simulink model "total_senario"  (R2019a)
settings: Solver=ode4  StartTime=0.0  StopTime=40  FixedStep=0.001  RelTol=1e-3
libraries: nesl_utility x16, sm_lib x13, simulink x1
(part 1 of 3)
settings Model: Creator=spring  LastModifiedBy=spring-dorosee

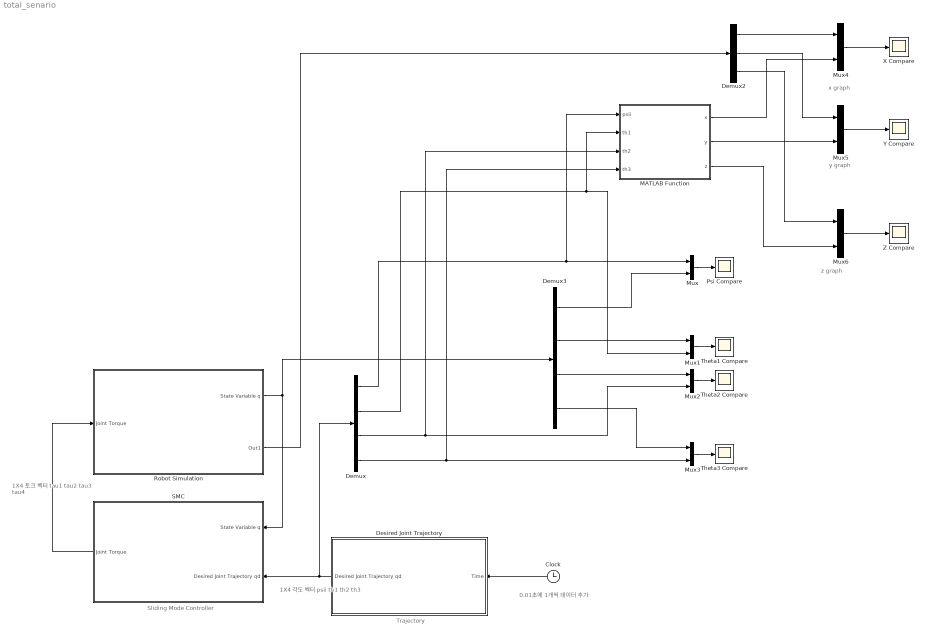
== system total_senario ==
  note: z graph
  note: y graph
  note: x graph
  note: 1X4 각도 벡터
      | psii
      | th1
      | th2
      | th3
  note: 0.01초에 1개씩 데이터 추가
  note: Trajectory
  note: Sliding Mode Controller
  note: 1X4 토크 벡터
      | tau1
      | tau2
      | tau3
      | tau4
  Clock : Clock
  Demux : Demux
  Demux2 : Demux  Outputs=3
  Demux3 : Demux
  Desired Joint Trajectory : Subsystem
  MATLAB Function : MATLAB Function  TreatAsAtomicUnit=on
  Mux{,1..6} (7 alike) : Mux  Inputs=2
  Psi Compare : Scope
  Robot Simulation : Subsystem
  SMC : Subsystem
  Theta1 Compare : Scope
  Theta2 Compare : Scope
  Theta3 Compare : Scope
  X Compare : Scope
  Y Compare : Scope
  Z Compare : Scope
  wires:
  SMC/1(Joint Torque) -> Robot Simulation/1(Joint Torque)
  Robot Simulation/1(State Variable q) -> SMC/1(State Variable q), Demux3/1
  Demux/1 -> MATLAB Function/1(psii), Mux/1
  Demux/2 -> Mux1/2, MATLAB Function/2(th1)
  Demux/3 -> Mux2/2, MATLAB Function/3(th2)
  Demux/4 -> Mux3/2, MATLAB Function/4(th3)
  Clock/1 -> Desired Joint Trajectory/1(Time)
  Desired Joint Trajectory/1(Desired Joint Trajectory qd) -> SMC/2(Desired Joint Trajectory qd), Demux/1
  Demux3/1 -> Mux/2
  Demux3/2 -> Mux1/1
  Demux3/3 -> Mux2/1
  Demux3/4 -> Mux3/1
  Mux/1 -> Psi Compare/1
  Mux1/1 -> Theta1 Compare/1
  Mux3/1 -> Theta3 Compare/1
  Mux2/1 -> Theta2 Compare/1
  Robot Simulation/2(Out1) -> Demux2/1
  Demux2/1 -> Mux4/1
  Demux2/2 -> Mux5/1
  MATLAB Function/1(x) -> Mux4/2
  MATLAB Function/2(y) -> Mux5/2
  Mux5/1 -> Y Compare/1
  Mux4/1 -> X Compare/1
  Demux2/3 -> Mux6/1
  MATLAB Function/3(z) -> Mux6/2
  Mux6/1 -> Z Compare/1

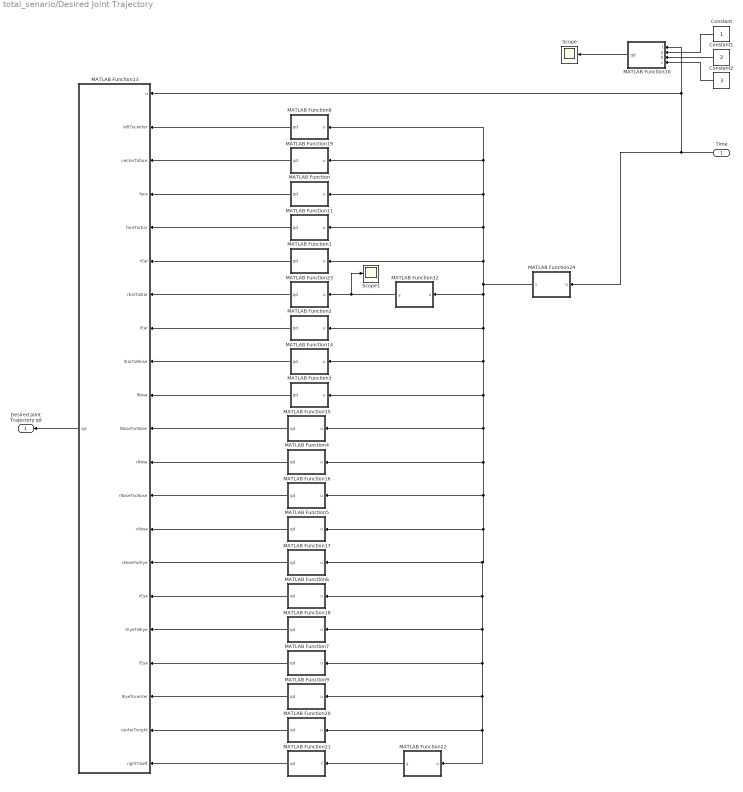
== system total_senario/Desired Joint Trajectory ==
  Time : Inport
  Constant : Constant
  Constant1 : Constant  Value=2
  Constant2 : Constant  Value=3
  MATLAB Function : MATLAB Function  TreatAsAtomicUnit=on
  MATLAB Function1 : MATLAB Function  TreatAsAtomicUnit=on
  MATLAB Function10 : MATLAB Function  TreatAsAtomicUnit=on
  MATLAB Function11 : MATLAB Function  TreatAsAtomicUnit=on
  MATLAB Function12 : MATLAB Function  TreatAsAtomicUnit=on
  MATLAB Function13 : MATLAB Function  TreatAsAtomicUnit=on
  MATLAB Function14 : MATLAB Function  TreatAsAtomicUnit=on
  MATLAB Function15 : MATLAB Function  TreatAsAtomicUnit=on
  MATLAB Function16 : MATLAB Function  TreatAsAtomicUnit=on
  MATLAB Function17 : MATLAB Function  TreatAsAtomicUnit=on
  MATLAB Function18 : MATLAB Function  TreatAsAtomicUnit=on
  MATLAB Function19 : MATLAB Function  TreatAsAtomicUnit=on
  MATLAB Function2 : MATLAB Function  TreatAsAtomicUnit=on
  MATLAB Function20 : MATLAB Function  TreatAsAtomicUnit=on
  MATLAB Function21 : MATLAB Function  TreatAsAtomicUnit=on
  MATLAB Function22 : MATLAB Function  TreatAsAtomicUnit=on
  MATLAB Function23 : MATLAB Function  TreatAsAtomicUnit=on
  MATLAB Function24 : MATLAB Function  TreatAsAtomicUnit=on
  MATLAB Function3 : MATLAB Function  TreatAsAtomicUnit=on
  MATLAB Function4 : MATLAB Function  TreatAsAtomicUnit=on
  MATLAB Function5 : MATLAB Function  TreatAsAtomicUnit=on
  MATLAB Function6 : MATLAB Function  TreatAsAtomicUnit=on
  MATLAB Function7 : MATLAB Function  TreatAsAtomicUnit=on
  MATLAB Function8 : MATLAB Function  TreatAsAtomicUnit=on
  MATLAB Function9 : MATLAB Function  TreatAsAtomicUnit=on
  Scope : Scope
  Scope1 : Scope
  Desired Joint Trajectory qd : Outport
  wires:
  MATLAB Function13/1(qd) -> Desired Joint Trajectory qd/1
  MATLAB Function10/1(qd) -> Scope/1
  Constant/1 -> MATLAB Function10/2(a)
  Constant1/1 -> MATLAB Function10/3(b)
  Constant2/1 -> MATLAB Function10/4(c)
  MATLAB Function19/1(qd) -> MATLAB Function13/3(centerToface)
  MATLAB Function/1(qd) -> MATLAB Function13/4(face)
  MATLAB Function11/1(qd) -> MATLAB Function13/5(faceTorEar)
  MATLAB Function1/1(qd) -> MATLAB Function13/6(rEar)
  MATLAB Function2/1(qd) -> MATLAB Function13/8(lEar)
  MATLAB Function14/1(qd) -> MATLAB Function13/9(lEarTolNose)
  MATLAB Function3/1(qd) -> MATLAB Function13/10(lNose)
  MATLAB Function15/1(qd) -> MATLAB Function13/11(lNoseTorNose)
  MATLAB Function4/1(qd) -> MATLAB Function13/12(rNose)
  MATLAB Function16/1(qd) -> MATLAB Function13/13(rNoseTocNose)
  MATLAB Function5/1(qd) -> MATLAB Function13/14(cNose)
  MATLAB Function17/1(qd) -> MATLAB Function13/15(cNoseTorEye)
  MATLAB Function6/1(qd) -> MATLAB Function13/16(rEye)
  MATLAB Function18/1(qd) -> MATLAB Function13/17(rEyeTolEye)
  MATLAB Function7/1(qd) -> MATLAB Function13/18(lEye)
  MATLAB Function8/1(qd) -> MATLAB Function13/2(leftTocenter)
  MATLAB Function9/1(qd) -> MATLAB Function13/19(lEyeTocenter)
  MATLAB Function20/1(qd) -> MATLAB Function13/20(centerToright)
  MATLAB Function21/1(qd) -> MATLAB Function13/21(rightToleft)
  MATLAB Function23/1(qd) -> MATLAB Function13/7(rEarTolEar)
  MATLAB Function12/1(y) -> Scope1/1, MATLAB Function23/1(u)
  MATLAB Function22/1(y) -> MATLAB Function21/1(t)
  Time/1 -> MATLAB Function24/1(u), MATLAB Function13/1(u), MATLAB Function10/1(t)
  MATLAB Function24/1(s) -> MATLAB Function1/1(u), MATLAB Function11/1(u), MATLAB Function/1(u), MATLAB Function19/1(u), MATLAB Function8/1(u), MATLAB Function22/1(u), MATLAB Function20/1(u), MATLAB Function9/1(u), MATLAB Function7/1(u), MATLAB Function18/1(u), MATLAB Function6/1(u), MATLAB Function17/1(u), MATLAB Function5/1(u), MATLAB Function16/1(u), MATLAB Function4/1(u), MATLAB Function15/1(u), MATLAB Function3/1(u), MATLAB Function14/1(u), MATLAB Function2/1(u), MATLAB Function12/1(u)

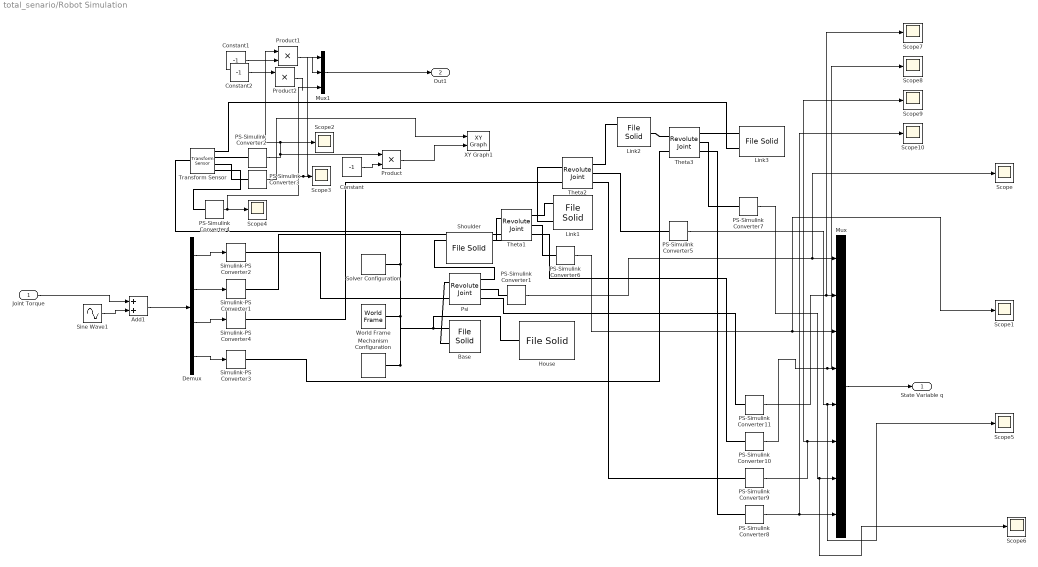
== system total_senario/Robot Simulation ==
  Joint Torque : Inport
  Add1 : Sum
  Base : sm_lib/Body Elements/File Solid  ExtGeomFileName=/Users/spring-dorosee/Desktop/project/inha/2학년 부분학기/로봇공학/로보트롤스/modeling/RotateBase.step  UnitType=FromFile  ExtGeomFileUnits=m  InertiaType=CalculateFromGeometry  Mass=2.945  MassUnits=kg  CenterOfMass=[0 0 0]  CenterOfMassUnits=m  MomentsOfInertia=[1 1 1]  MomentsOfInertiaUnits=kg*m^2  ProductsOfInertia=[0 0 0]  ProductsOfInertiaUnits=kg*m^2  BasedOnType=Density  Density=1000  DensityUnits=kg/m^3  DoExposeReferenceFrame=on  SerializedFrames=<Frames><Frame><Id>Frame1</Id><Value><Name>BaseFrame</Name><Origin><Source>GeometricFeature</Source><FeatureName>planar surface 2</FeatureName></Origin><PrimaryAxis><DefinedDirection>+Z</DefinedDirection><Source>ReferenceFrame</Source><SourceDirection>+Z</SourceDirection><FeatureName></FeatureName></PrimaryAxis><SecondaryAxis><DefinedDirection>+X</DefinedDirection><Source>ReferenceFrame</Source><SourceDirection>+X</SourceDirection><FeatureName></FeatureName></SecondaryAxis></Value></Frame><Frame><Id>Frame2</Id><Value><Name>Shoulder</Name><Origin><Source>GeometricFeature</Source><FeatureName>planar surface 1</FeatureName></Origin><PrimaryAxis><DefinedDirection>+Z</DefinedDirection><Source>ReferenceFrame</Source><SourceDirection>+Z</SourceDirection><FeatureName></FeatureName></PrimaryAxis><SecondaryAxis><DefinedDirection>+X</DefinedDirection><Source>ReferenceFrame</Source><SourceDirection>+X</SourceDirection><FeatureName></FeatureName></SecondaryAxis></Value></Frame></Frames>  GraphicType=FromGeometry  MarkerShape=Sphere  MarkerSize=10  GraphicVisPropType=SimpleVisualProperties  GraphicDiffuseColor=[0.0 0.8 0.8]  GraphicSpecularColor=[0.5 0.5 0.5 1.0]  GraphicAmbientColor=[0.15 0.15 0.15 1.0]  GraphicEmissiveColor=[0.0 0.0 0.0 1.0]  GraphicShininess=75  GraphicOpacity=1.0
  Constant : Constant  Value=-1
  Constant1 : Constant  Value=-1
  Constant2 : Constant  Value=-1
  Demux : Demux
  House : sm_lib/Body Elements/File Solid  ExtGeomFileName=C:\Users\Hyeong Deok Seo\Desktop\robot_matlab\deok\robot_team\simul\house.step  UnitType=FromFile  ExtGeomFileUnits=m  InertiaType=Custom  Mass=0.1  MassUnits=kg  CenterOfMass=[0 0 0.08]  CenterOfMassUnits=m  MomentsOfInertia=[1 1 1]  MomentsOfInertiaUnits=kg*m^2  ProductsOfInertia=[0 0 0]  ProductsOfInertiaUnits=kg*m^2  BasedOnType=Density  Density=1000  DensityUnits=kg/m^3  DoExposeReferenceFrame=off  SerializedFrames=<Frames><Frame><Id>Frame1</Id><Value><Name>BaseFrame</Name><Origin><Source>GeometricFeature</Source><FeatureName>planar surface 7</FeatureName></Origin><PrimaryAxis><DefinedDirection>+Z</DefinedDirection><Source>ReferenceFrame</Source><SourceDirection>+Z</SourceDirection><FeatureName></FeatureName></PrimaryAxis><SecondaryAxis><DefinedDirection>+X</DefinedDirection><Source>GeometricFeature</Source><SourceDirection>+X</SourceDirection><FeatureName>planar surface 4</FeatureName></SecondaryAxis></Value></Frame></Frames>  GraphicType=FromGeometry  MarkerShape=Sphere  MarkerSize=10  GraphicVisPropType=SimpleVisualProperties  GraphicDiffuseColor=[1.0 1.0 0.2]  GraphicSpecularColor=[0.5 0.5 0.5 1.0]  GraphicAmbientColor=[0.15 0.15 0.15 1.0]  GraphicEmissiveColor=[0.0 0.0 0.0 1.0]  GraphicShininess=75  GraphicOpacity=1.0
  Link1 : sm_lib/Body Elements/File Solid  ExtGeomFileName=/Users/spring-dorosee/Desktop/project/inha/2학년 부분학기/로봇공학/로보트롤스/modeling/link1_30cm.step  UnitType=FromFile  ExtGeomFileUnits=m  InertiaType=Custom  Mass=4  MassUnits=kg  CenterOfMass=[0 0 0.38]  CenterOfMassUnits=m  MomentsOfInertia=[0 0 0]  MomentsOfInertiaUnits=kg*m^2  ProductsOfInertia=[0 0 0]  ProductsOfInertiaUnits=kg*m^2  BasedOnType=Density  Density=1000  DensityUnits=kg/m^3  DoExposeReferenceFrame=on  SerializedFrames=<Frames><Frame><Id>Frame1</Id><Value><Name>Theta1</Name><Origin><Source>GeometricFeature</Source><FeatureName>planar surface 2</FeatureName></Origin><PrimaryAxis><DefinedDirection>+X</DefinedDirection><Source>ReferenceFrame</Source><SourceDirection>+Z</SourceDirection><FeatureName></FeatureName></PrimaryAxis><SecondaryAxis><DefinedDirection>+Z</DefinedDirection><Source>ReferenceFrame</Source><SourceDirection>+X</SourceDirection><FeatureName></FeatureName></SecondaryAxis></Value></Frame><Frame><Id>Frame2</Id><Value><Name>Theta2</Name><Origin><Source>CenterOfMassFrame</Source><FeatureName></FeatureName></Origin><PrimaryAxis><DefinedDirection>+X</DefinedDirection><Source>ReferenceFrame</Source><SourceDirection>+Z</SourceDirection><FeatureName></FeatureName></PrimaryAxis><SecondaryAxis><DefinedDirection>+Z</DefinedDirection><Source>ReferenceFrame</Source><SourceDirection>+X</SourceDirection><FeatureName></FeatureName></SecondaryAxis></Value></Frame></Frames>  GraphicType=FromGeometry  MarkerShape=Sphere  MarkerSize=10  GraphicVisPropType=SimpleVisualProperties  GraphicDiffuseColor=[0.6 0.6 1.0]  GraphicSpecularColor=[0.5 0.5 0.5 1.0]  GraphicAmbientColor=[0.15 0.15 0.15 1.0]  GraphicEmissiveColor=[0.0 0.0 0.0 1.0]  GraphicShininess=75  GraphicOpacity=1.0
  Link2 : sm_lib/Body Elements/File Solid  ExtGeomFileName=/Users/spring-dorosee/Desktop/project/inha/2학년 부분학기/로봇공학/로보트롤스/modeling/link1_30cm.step  UnitType=FromFile  ExtGeomFileUnits=m  InertiaType=Custom  Mass=3  MassUnits=kg  CenterOfMass=[0 0 0.38]  CenterOfMassUnits=m  MomentsOfInertia=[0 0 0]  MomentsOfInertiaUnits=kg*m^2  ProductsOfInertia=[0 0 0]  ProductsOfInertiaUnits=kg*m^2  BasedOnType=Density  Density=1000  DensityUnits=kg/m^3  DoExposeReferenceFrame=off  SerializedFrames=<Frames><Frame><Id>Frame1</Id><Value><Name>Theta2</Name><Origin><Source>GeometricFeature</Source><FeatureName>planar surface 2</FeatureName></Origin><PrimaryAxis><DefinedDirection>+X</DefinedDirection><Source>ReferenceFrame</Source><SourceDirection>+Z</SourceDirection><FeatureName></FeatureName></PrimaryAxis><SecondaryAxis><DefinedDirection>+Z</DefinedDirection><Source>ReferenceFrame</Source><SourceDirection>+X</SourceDirection><FeatureName></FeatureName></SecondaryAxis></Value></Frame><Frame><Id>Frame2</Id><Value><Name>Theta3</Name><Origin><Source>CenterOfMassFrame</Source><FeatureName></FeatureName></Origin><PrimaryAxis><DefinedDirection>+X</DefinedDirection><Source>ReferenceFrame</Source><SourceDirection>+Z</SourceDirection><FeatureName></FeatureName></PrimaryAxis><SecondaryAxis><DefinedDirection>+Z</DefinedDirection><Source>ReferenceFrame</Source><SourceDirection>+X</SourceDirection><FeatureName></FeatureName></SecondaryAxis></Value></Frame><Frame><Id>Frame3</Id><Value><Name>XYZ</Name><Origin><Source>GeometricFeature</Source><FeatureName>cylindrical surface 7</FeatureName></Origin><PrimaryAxis><DefinedDirection>+X</DefinedDirection><Source>ReferenceFrame</Source><SourceDirection>+Z</SourceDirection><FeatureName></FeatureName></PrimaryAxis><SecondaryAxis><DefinedDirection>+Z</DefinedDirection><Source>ReferenceFrame</Source><SourceDirection>+X</SourceDirection><FeatureName></FeatureName></SecondaryAxis></Value></Frame></Frames>  GraphicType=FromGeometry  MarkerShape=Sphere  MarkerSize=10  GraphicVisPropType=SimpleVisualProperties  GraphicDiffuseColor=[1.0 0.6 0.6]  GraphicSpecularColor=[0.5 0.5 0.5 1.0]  GraphicAmbientColor=[0.15 0.15 0.15 1.0]  GraphicEmissiveColor=[0.0 0.0 0.0 1.0]  GraphicShininess=75  GraphicOpacity=1.0
  Link3 : sm_lib/Body Elements/File Solid  ExtGeomFileName=/Users/spring-dorosee/Desktop/project/inha/2학년 부분학기/로봇공학/로보트롤스/modeling/WafflePlate.step  UnitType=FromFile  ExtGeomFileUnits=m  InertiaType=Custom  Mass=1  MassUnits=kg  CenterOfMass=[0 0 0.856]  CenterOfMassUnits=m  MomentsOfInertia=[0 0 0]  MomentsOfInertiaUnits=kg*m^2  ProductsOfInertia=[0 0 0]  ProductsOfInertiaUnits=kg*m^2  BasedOnType=Density  Density=1000  DensityUnits=kg/m^3  DoExposeReferenceFrame=on  SerializedFrames=<Frames><Frame><Id>Frame1</Id><Value><Name>Theta3</Name><Origin><Source>GeometricFeature</Source><FeatureName>planar surface 1</FeatureName></Origin><PrimaryAxis><DefinedDirection>+X</DefinedDirection><Source>ReferenceFrame</Source><SourceDirection>+Z</SourceDirection><FeatureName></FeatureName></PrimaryAxis><SecondaryAxis><DefinedDirection>+Z</DefinedDirection><Source>ReferenceFrame</Source><SourceDirection>+X</SourceDirection><FeatureName></FeatureName></SecondaryAxis></Value></Frame><Frame><Id>Frame2</Id><Value><Name>CenterMass</Name><Origin><Source>CenterOfMassFrame</Source><FeatureName></FeatureName></Origin><PrimaryAxis><DefinedDirection>+Z</DefinedDirection><Source>ReferenceFrame</Source><SourceDirection>+Z</SourceDirection><FeatureName></FeatureName></PrimaryAxis><SecondaryAxis><DefinedDirection>+X</DefinedDirection><Source>ReferenceFrame</Source><SourceDirection>+X</SourceDirection><FeatureName></FeatureName></SecondaryAxis></Value></Frame></Frames>  GraphicType=FromGeometry  MarkerShape=Sphere  MarkerSize=10  GraphicVisPropType=SimpleVisualProperties  GraphicDiffuseColor=[0.4 1.0 0.4]  GraphicSpecularColor=[0.5 0.5 0.5 1.0]  GraphicAmbientColor=[0.15 0.15 0.15 1.0]  GraphicEmissiveColor=[0.0 0.0 0.0 1.0]  GraphicShininess=75  GraphicOpacity=1.0
  Mechanism Configuration : sm_lib/Utilities/Mechanism Configuration  UniformGravity=Constant  GravityVector=[0 0 -9.81]  GravityUnits=m/s^2  LinearizationDelta=0.001
  Mux : Mux  Inputs=8
  Mux1 : Mux  Inputs=3
  PS-Simulink Converter{1..11} (11 alike) : nesl_utility/PS-Simulink Converter  PhysicalDomain=network_engine_domain  SubClassName=ps_output  LeftPortType=input  RightPortType=output  PseudoPeriodic=off  Frequencies=[]  Unit=1  AffineConversion=off
      settings: SourceProductBaseCode=PW,SS
  Product : Product
  Product1 : Product
  Product2 : Product
  Psi : sm_lib/Joints/Revolute Joint  SenseConstraintForce=off  SenseConstraintForceX=off  SenseConstraintForceY=off  SenseConstraintForceZ=off  SenseConstraintTorque=off  SenseConstraintTorqueX=off  SenseConstraintTorqueY=off  SenseConstraintTorqueZ=off  SenseTotalForce=off  SenseTotalForceX=off  SenseTotalForceY=off  SenseTotalForceZ=off  SenseTotalTorque=off  SenseTotalTorqueX=off  SenseTotalTorqueY=off  SenseTotalTorqueZ=off  CompositeWrenchDir=FollowerOnBase  CompositeWrenchFrame=BaseFrame  EquilibriumPosition=0  EquilibriumPositionUnits=deg  SpringStiffness=0  SpringStiffnessUnits=N*m/deg  DampingCoefficient=0  DampingCoefficientUnits=N*m/(deg/s)  TorqueActuationMode=InputTorque  MotionActuationMode=ComputedMotion  SensePosition=on  SenseVelocity=on  SenseAcceleration=off  SenseTorqueForce=off  SenseLowerLimitTorqueForce=off  SenseUpperLimitTorqueForce=off  LowerLimitSpecify=off  LowerLimitBound=-90  LowerLimitBoundUnits=deg  LowerLimitStiffness=1e4  LowerLimitStiffnessUnits=N*m/deg  LowerLimitDamping=10  LowerLimitDampingUnits=N*m/(deg/s)  LowerLimitTransitionRegionWidth=0.1  LowerLimitTransitionRegionWidthUnits=deg  UpperLimitSpecify=off  UpperLimitBound=90  UpperLimitBoundUnits=deg  UpperLimitStiffness=1e4  UpperLimitStiffnessUnits=N*m/deg  UpperLimitDamping=10  UpperLimitDampingUnits=N*m/(deg/s)  UpperLimitTransitionRegionWidth=0.1  UpperLimitTransitionRegionWidthUnits=deg  PositionTargetSpecify=on  PositionTargetPriority=High  PositionTargetValue=2.3562  PositionTargetValueUnits=rad  VelocityTargetSpecify=on  VelocityTargetPriority=High  VelocityTargetValue=0  VelocityTargetValueUnits=deg/s
  Scope{,1..10} (11 alike) : Scope
  Shoulder : sm_lib/Body Elements/File Solid  ExtGeomFileName=/Users/spring-dorosee/Desktop/project/inha/2학년 부분학기/로봇공학/로보트롤스/modeling/Shoulder.step  UnitType=FromFile  ExtGeomFileUnits=m  InertiaType=Custom  Mass=500  MassUnits=kg  CenterOfMass=[0 0 0.08]  CenterOfMassUnits=m  MomentsOfInertia=[0 0 0]  MomentsOfInertiaUnits=kg*m^2  ProductsOfInertia=[0 0 0]  ProductsOfInertiaUnits=kg*m^2  BasedOnType=Density  Density=1000  DensityUnits=kg/m^3  DoExposeReferenceFrame=on  SerializedFrames=<Frames><Frame><Id>Frame1</Id><Value><Name>Theta1</Name><Origin><Source>CenterOfMassFrame</Source><FeatureName></FeatureName></Origin><PrimaryAxis><DefinedDirection>+Y</DefinedDirection><Source>ReferenceFrame</Source><SourceDirection>+Z</SourceDirection><FeatureName></FeatureName></PrimaryAxis><SecondaryAxis><DefinedDirection>+Z</DefinedDirection><Source>ReferenceFrame</Source><SourceDirection>+X</SourceDirection><FeatureName></FeatureName></SecondaryAxis></Value></Frame><Frame><Id>Frame2</Id><Value><Name>ShoulderFrame</Name><Origin><Source>CenterOfMassFrame</Source><FeatureName></FeatureName></Origin><PrimaryAxis><DefinedDirection>+Z</DefinedDirection><Source>ReferenceFrame</Source><SourceDirection>+Z</SourceDirection><FeatureName></FeatureName></PrimaryAxis><SecondaryAxis><DefinedDirection>+X</DefinedDirection><Source>ReferenceFrame</Source><SourceDirection>+X</SourceDirection><FeatureName></FeatureName></SecondaryAxis></Value></Frame><Frame><Id>Frame3</Id><Value><Name>F3</Name><Origin><Source>CenterOfMassFrame</Source><FeatureName></FeatureName></Origin><PrimaryAxis><DefinedDirection>+Z</DefinedDirection><Source>ReferenceFrame</Source><SourceDirection>+Z</SourceDirection><FeatureName></FeatureName></PrimaryAxis><SecondaryAxis><DefinedDirection>+X</DefinedDirection><Source>ReferenceFrame</Source><SourceDirection>+X</SourceDirection><FeatureName></FeatureName></SecondaryAxis></Value></Frame></Frames>  GraphicType=FromGeometry  MarkerShape=Sphere  MarkerSize=10  GraphicVisPropType=SimpleVisualProperties  GraphicDiffuseColor=[1.0 1.0 0.2]  GraphicSpecularColor=[0.5 0.5 0.5 1.0]  GraphicAmbientColor=[0.15 0.15 0.15 1.0]  GraphicEmissiveColor=[0.0 0.0 0.0 1.0]  GraphicShininess=75  GraphicOpacity=1.0
  Simulink-PS Converter{1..4} (4 alike) : nesl_utility/Simulink-PS Converter  PhysicalDomain=network_engine_domain  SubClassName=ps_input  LeftPortType=input  RightPortType=output  PseudoPeriodic=off  Frequencies=[]  NoiseDistribution=none  NoiseParameters=[]  Unit=1  AffineConversion=off  FilteringAndDerivatives=filter  SimscapeFilterOrder=2  InputFilterTimeConstant=0.001  UdotUserProvided=1
      settings: SourceProductBaseCode=PW,SS
  Sine Wave1 : Sin  Amplitude=0.1  SampleTime=0
  Solver Configuration : nesl_utility/Solver Configuration  PhysicalDomain=network_engine_domain  SubClassName=solver  LeftPortType=input  RightPortType=generic  Tones=[]  Harmonics=[]  SimulateNoise=off  Profile=off  UseLocalSampling=off  EnableSwitchedLinearOptims=on  FrequencyDomain=off  UseCCode=off  RelTol=0.001  AbsTol=1e-06  MinStep=1e-09  ToWorkspace=off  RevertToSquareIcSolve=off  NumHomotopyIterations=100  PhasorMode=off  PhasorModeNumHarmonics=1  DoDC=off  ResidualTolerance=1e-09  UseLocalSolver=off  LocalSolverChoice=NE_BACKWARD_EULER_ADVANCER  LocalSolverSampleTime=0.001  DoFixedCost=off  MaxNonlinIter=3  MaxModeIter=2  LinearAlgebra=Sparse  EquationFormulation=NE_TIME_EF  DelaysMemoryBudget=1024  AutomaticFiltering=on  FilteringTimeConstant=0.001  PartitionStorageMethod=AS_NEEDED  PartitionMemoryBudget=1024  PartitionMethod=FAST
      settings: SourceProductBaseCode=PW,SS
  Theta1 : sm_lib/Joints/Revolute Joint  SenseConstraintForce=off  SenseConstraintForceX=off  SenseConstraintForceY=off  SenseConstraintForceZ=off  SenseConstraintTorque=off  SenseConstraintTorqueX=off  SenseConstraintTorqueY=off  SenseConstraintTorqueZ=off  SenseTotalForce=off  SenseTotalForceX=off  SenseTotalForceY=off  SenseTotalForceZ=off  SenseTotalTorque=off  SenseTotalTorqueX=off  SenseTotalTorqueY=off  SenseTotalTorqueZ=off  CompositeWrenchDir=FollowerOnBase  CompositeWrenchFrame=BaseFrame  EquilibriumPosition=0  EquilibriumPositionUnits=deg  SpringStiffness=0  SpringStiffnessUnits=N*m/deg  DampingCoefficient=0  DampingCoefficientUnits=N*m/(deg/s)  TorqueActuationMode=InputTorque  MotionActuationMode=ComputedMotion  SensePosition=on  SenseVelocity=on  SenseAcceleration=off  SenseTorqueForce=off  SenseLowerLimitTorqueForce=off  SenseUpperLimitTorqueForce=off  LowerLimitSpecify=off  LowerLimitBound=-90  LowerLimitBoundUnits=deg  LowerLimitStiffness=1e4  LowerLimitStiffnessUnits=N*m/deg  LowerLimitDamping=10  LowerLimitDampingUnits=N*m/(deg/s)  LowerLimitTransitionRegionWidth=0.1  LowerLimitTransitionRegionWidthUnits=deg  UpperLimitSpecify=off  UpperLimitBound=90  UpperLimitBoundUnits=deg  UpperLimitStiffness=1e4  UpperLimitStiffnessUnits=N*m/deg  UpperLimitDamping=10  UpperLimitDampingUnits=N*m/(deg/s)  UpperLimitTransitionRegionWidth=0.1  UpperLimitTransitionRegionWidthUnits=deg  PositionTargetSpecify=on  PositionTargetPriority=High  PositionTargetValue=-0.7249  PositionTargetValueUnits=rad  VelocityTargetSpecify=on  VelocityTargetPriority=High  VelocityTargetValue=0  VelocityTargetValueUnits=deg/s
  Theta2 : sm_lib/Joints/Revolute Joint  SenseConstraintForce=off  SenseConstraintForceX=off  SenseConstraintForceY=off  SenseConstraintForceZ=off  SenseConstraintTorque=off  SenseConstraintTorqueX=off  SenseConstraintTorqueY=off  SenseConstraintTorqueZ=off  SenseTotalForce=off  SenseTotalForceX=off  SenseTotalForceY=off  SenseTotalForceZ=off  SenseTotalTorque=off  SenseTotalTorqueX=off  SenseTotalTorqueY=off  SenseTotalTorqueZ=off  CompositeWrenchDir=FollowerOnBase  CompositeWrenchFrame=BaseFrame  EquilibriumPosition=0  EquilibriumPositionUnits=deg  SpringStiffness=0  SpringStiffnessUnits=N*m/deg  DampingCoefficient=0  DampingCoefficientUnits=N*m/(deg/s)  TorqueActuationMode=InputTorque  MotionActuationMode=ComputedMotion  SensePosition=on  SenseVelocity=on  SenseAcceleration=off  SenseTorqueForce=off  SenseLowerLimitTorqueForce=off  SenseUpperLimitTorqueForce=off  LowerLimitSpecify=off  LowerLimitBound=-90  LowerLimitBoundUnits=deg  LowerLimitStiffness=1e4  LowerLimitStiffnessUnits=N*m/deg  LowerLimitDamping=10  LowerLimitDampingUnits=N*m/(deg/s)  LowerLimitTransitionRegionWidth=0.1  LowerLimitTransitionRegionWidthUnits=deg  UpperLimitSpecify=off  UpperLimitBound=90  UpperLimitBoundUnits=deg  UpperLimitStiffness=1e4  UpperLimitStiffnessUnits=N*m/deg  UpperLimitDamping=10  UpperLimitDampingUnits=N*m/(deg/s)  UpperLimitTransitionRegionWidth=0.1  UpperLimitTransitionRegionWidthUnits=deg  PositionTargetSpecify=on  PositionTargetPriority=High  PositionTargetValue=1.1324  PositionTargetValueUnits=rad  VelocityTargetSpecify=on  VelocityTargetPriority=High  VelocityTargetValue=0  VelocityTargetValueUnits=deg/s
  Theta3 : sm_lib/Joints/Revolute Joint  SenseConstraintForce=off  SenseConstraintForceX=off  SenseConstraintForceY=off  SenseConstraintForceZ=off  SenseConstraintTorque=off  SenseConstraintTorqueX=off  SenseConstraintTorqueY=off  SenseConstraintTorqueZ=off  SenseTotalForce=off  SenseTotalForceX=off  SenseTotalForceY=off  SenseTotalForceZ=off  SenseTotalTorque=off  SenseTotalTorqueX=off  SenseTotalTorqueY=off  SenseTotalTorqueZ=off  CompositeWrenchDir=FollowerOnBase  CompositeWrenchFrame=BaseFrame  EquilibriumPosition=0  EquilibriumPositionUnits=deg  SpringStiffness=0  SpringStiffnessUnits=N*m/deg  DampingCoefficient=0  DampingCoefficientUnits=N*m/(deg/s)  TorqueActuationMode=InputTorque  MotionActuationMode=ComputedMotion  SensePosition=on  SenseVelocity=on  SenseAcceleration=off  SenseTorqueForce=off  SenseLowerLimitTorqueForce=off  SenseUpperLimitTorqueForce=off  LowerLimitSpecify=off  LowerLimitBound=-90  LowerLimitBoundUnits=deg  LowerLimitStiffness=1e4  LowerLimitStiffnessUnits=N*m/deg  LowerLimitDamping=10  LowerLimitDampingUnits=N*m/(deg/s)  LowerLimitTransitionRegionWidth=0.1  LowerLimitTransitionRegionWidthUnits=deg  UpperLimitSpecify=off  UpperLimitBound=90  UpperLimitBoundUnits=deg  UpperLimitStiffness=1e4  UpperLimitStiffnessUnits=N*m/deg  UpperLimitDamping=10  UpperLimitDampingUnits=N*m/(deg/s)  UpperLimitTransitionRegionWidth=0.1  UpperLimitTransitionRegionWidthUnits=deg  PositionTargetSpecify=on  PositionTargetPriority=High  PositionTargetValue=1.163296326794896  PositionTargetValueUnits=rad  VelocityTargetSpecify=on  VelocityTargetPriority=High  VelocityTargetValue=0  VelocityTargetValueUnits=deg/s
  Transform Sensor : sm_lib/Frames and Transforms/Transform Sensor  MeasurementFrame=World  SenseAngle=off  SenseAxis=off  SenseAngle1=off  SenseAngle2=off  SenseAngle3=off  SenseQ=off  SenseR=off  SenseOmegaX=off  SenseOmegaY=off  SenseOmegaZ=off  SenseOmega1=off  SenseOmega2=off  SenseOmega3=off  SenseQDot=off  SenseRDot=off  SenseAlphaX=off  SenseAlphaY=off  SenseAlphaZ=off  SenseAlpha1=off  SenseAlpha2=off  SenseAlpha3=off  SenseQDDot=off  SenseRDDot=off  SenseX=on  SenseY=on  SenseZ=on  SenseRad=off  SenseAzim=off  SenseDist=off  SenseInc=off  SenseXDot=off  SenseYDot=off  SenseZDot=off  SenseRadDot=off  SenseAzimDot=off  SenseDistDot=off  SenseIncDot=off  SenseXDDot=off  SenseYDDot=off  SenseZDDot=off  SenseRadDDot=off  SenseAzimDDot=off  SenseDistDDot=off  SenseIncDDot=off
  World Frame : sm_lib/Frames and Transforms/World Frame
  XY Graph1 : simulink/Sinks/XY Graph  xmin=-0.4  xmax=0.4  ymin=0  ymax=0.6  st=-1
  State Variable q : Outport
  Out1 : Outport  Port=2
  wires:
  PS-Simulink Converter7/1 -> Scope6/1, Mux/7
  Product/1 -> XY Graph1/2
  Constant/1 -> Product/2
  PS-Simulink Converter4/1 -> Mux1/3, Scope4/1
  PS-Simulink Converter1/1 -> Scope/1, Mux/1
  PS-Simulink Converter6/1 -> Scope1/1, Mux/3
  PS-Simulink Converter5/1 -> Scope5/1, Mux/5
  PS-Simulink Converter2/1 -> Product/1, Scope2/1, Product1/1
  PS-Simulink Converter3/1 -> XY Graph1/1, Mux1/1, Scope3/1
  Demux/1 -> Simulink-PS Converter2/1
  Demux/2 -> Simulink-PS Converter1/1
  Demux/3 -> Simulink-PS Converter4/1
  Demux/4 -> Simulink-PS Converter3/1
  Mux/1 -> State Variable q/1
  PS-Simulink Converter10/1 -> Scope8/1, Mux/4
  PS-Simulink Converter9/1 -> Mux/6, Scope9/1
  PS-Simulink Converter8/1 -> Mux/8, Scope10/1
  PS-Simulink Converter11/1 -> Scope7/1, Mux/2
  Mux1/1 -> Out1/1
  Constant1/1 -> Product1/2
  Constant2/1 -> Product2/1
  Product2/1 -> ?
  Product1/1 -> Mux1/2
  Add1/1 -> Demux/1
  Joint Torque/1 -> Add1/1
  Sine Wave1/1 -> Add1/2
  connections:
  Shoulder/LConn1 -- Theta1/LConn1
  Theta3/LConn1 -- Link2/RConn1
  Psi/RConn1 -- Shoulder/RConn1
  Transform Sensor/RConn3 -- PS-Simulink Converter3/LConn1
  Theta3/RConn1 -- Link3/LConn1
  Simulink-PS Converter2/RConn1 -- Psi/LConn2
  Theta1/RConn1 -- Link1/LConn1
  Theta1/RConn2 -- PS-Simulink Converter6/LConn1
  Transform Sensor/RConn4 -- PS-Simulink Converter4/LConn1
  Theta3/LConn2 -- Simulink-PS Converter3/RConn1
  Link3/LConn2 -- Transform Sensor/RConn1
  Transform Sensor/RConn2 -- PS-Simulink Converter2/LConn1
  Theta1/LConn2 -- Simulink-PS Converter1/RConn1
  Psi/RConn2 -- PS-Simulink Converter1/LConn1
  Mechanism Configuration/RConn1 -- House/LConn1 -- Base/LConn1 -- Solver Configuration/RConn1 -- Transform Sensor/LConn1 -- World Frame/RConn1
  Theta3/RConn2 -- PS-Simulink Converter7/LConn1
  Theta2/RConn2 -- PS-Simulink Converter5/LConn1
  Base/LConn2 -- Psi/LConn1
  Link1/LConn2 -- Theta2/LConn1
  Theta2/RConn1 -- Link2/LConn1
  Simulink-PS Converter4/RConn1 -- Theta2/LConn2
  Psi/RConn3 -- PS-Simulink Converter11/LConn1
  Theta1/RConn3 -- PS-Simulink Converter10/LConn1
  Theta2/RConn3 -- PS-Simulink Converter9/LConn1
  Theta3/RConn3 -- PS-Simulink Converter8/LConn1

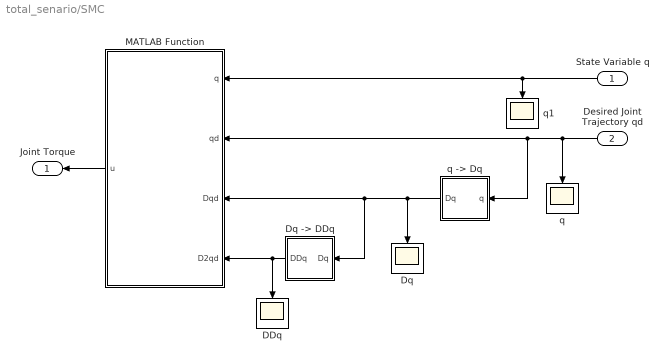
== system total_senario/SMC ==
  State Variable q : Inport
  Desired Joint Trajectory qd : Inport  Port=2
  DDq : Scope
  Dq : Scope
  "Dq -> DDq" : Subsystem
  MATLAB Function : MATLAB Function  TreatAsAtomicUnit=on
  q : Scope
  "q -> Dq" : Subsystem
  q1 : Scope
  Joint Torque : Outport
  wires:
  MATLAB Function/1(u) -> Joint Torque/1
  State Variable q/1 -> MATLAB Function/1(q), q1/1
  Desired Joint Trajectory qd/1 -> "q -> Dq"/1(q), MATLAB Function/2(qd), q/1
  "q -> Dq"/1(Dq) -> MATLAB Function/3(Dqd), "Dq -> DDq"/1(Dq), Dq/1
  "Dq -> DDq"/1(DDq) -> MATLAB Function/4(D2qd), DDq/1

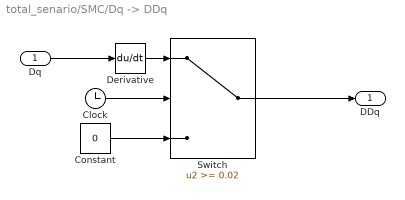
== system total_senario/SMC/Dq -> DDq ==
  Dq : Inport
  Clock : Clock
  Constant : Constant  Value=0
  Derivative : Derivative
  Switch : Switch  Threshold=0.02
  DDq : Outport
  wires:
  Switch/1 -> DDq/1
  Clock/1 -> Switch/2
  Constant/1 -> Switch/3
  Dq/1 -> Derivative/1
  Derivative/1 -> Switch/1

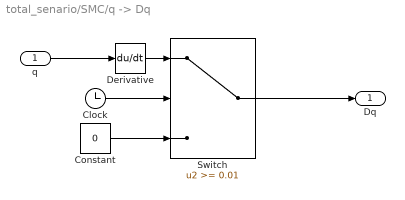
== system total_senario/SMC/q -> Dq ==
  q : Inport
  Clock : Clock
  Constant : Constant  Value=0
  Derivative : Derivative
  Switch : Switch  Threshold=0.01
  Dq : Outport
  wires:
  Derivative/1 -> Switch/1
  q/1 -> Derivative/1
  Constant/1 -> Switch/3
  Clock/1 -> Switch/2
  Switch/1 -> Dq/1

== matlab function total_senario/Desired Joint Trajectory/MATLAB Function1 ==
  data: u input; qd output

function qd = fcn(u)
t = u(1);
% time = 0:0.01:10

% (1) r_t,theta_t _ // for Tornado
% cycle=5; % 해당 시간동안 몇바퀴 돌지_진동수
% r_t = 0.1 - (0.1/tf)*t; 
% w_t = cycle*2*pi/tf; 
% theta_t = w_t*t;
% 
% % (2) waffle 중심 cartesian coordinate
% x_wa = r_t.*cos(theta_t); % waffle 중심  
% y_wa = r_t.*sin(theta_t) + 0.4;
% z_wa = - 0.2 - (0.3/tf)*t + 0.6; 
% r_wa = sqrt(x_wa.^2+y_wa.^2);

% psii= atan2(y_wa,x_wa);
% th2 = acos((r_wa.^2+z_wa.^2-L1^2-L2^2)./(2*L1*L2)); % r,z 좌표계로 사이드뷰
% th1 = atan2(z_wa-L3,r_wa) - atan2(L2*sin(th2),L1+L2*cos(th2));
% th3 = pi/2-th1-th2;

x = 0;
y = 0.4;

scale_factor = 1/80;
cycle = 1;
time = 1; %% 20
t=t/time;
w = 2*pi*cycle;
theta = w*t;


psii= psid(t);
th2 = th2d(t); % r,z 좌표계로 사이드뷰
th1 = th1d(t);
th3 = th3d(t);


qd = [psii; th1; th2; th3];

end

function y = s(t)
% if (-1<=t && t<3)
%     y = 2/3*t^3 - 8/27*t^4 +1/27*t^5;
% %     y = 3/2*t^3 - 1*t^4 +3/16*t^5; % 5 / 2
% %     y = 6*t^3 -8*t^4 + 3*t^5; % 5차 1초
% %     y = 2/3*t^2-1/9*t^3; % 3초
% %     y = t^2 - 0.25*t^3; % 2초
% %     y = 2*t^2 - t^3; % 1초
% %     y = t^2;
% elseif (3<=t && t<7)
%     y = t;
% elseif (7<=t &&  t<=10.01)
%     y = -37730/27 + 2600/3*t -5740/27*t^2 + 698/27*t^3 -14/9*t^4 + 1/27*t^5;
% %     y = -10240 + 5825*t -1320*t^2 + 149*t^3 -67/8*t^4 + 3/16*t^5; % 5 / 2
% %     y = -225990 + 119800*t -25380*t^2 + 2686*t^3 -142*t^4 + 3*t^5; % 5차1s
% %     y = 490/9 - 20*t + 8/3*t^2 - 1/9*t^3; % 3초
% %     y = 160 - 55*t +6.5 * t^2 - 0.25*t^3; % 2초
% %     y = 810 - 260*t + 28*t^2 - t^3; % 1초
% %     y = 10 - (t-10)^2;
% else
%     y=t;
% end
y = t;
end


function q = psid(t)

% global L1 L2 L3;
% q = 1.32;
q = atan2(yd(t),xd(t));
% q = 1.32;
end

function q = th1d(t)
L0=1.5;L1=0.3;L2=0.3;L3=0.08; % L3 항상 지면에 수직. 
tf=10; w = 10*pi/tf;
% global L1 L2 L3;
% q = -pi/6;
q = atan2(zd(t)-L3-1.5,sqrt(xd(t)^2+yd(t)^2)) - atan2(L2*sin(th2d(t)),L1+L2*cos(th2d(t)));
% q = -1.52;
end

function q = th2d(t)
L0=1.5;L1=0.3;L2=0.3;L3=0.08; % L3 항상 지면에 수직. 
tf=10; w = 10*pi/tf;
% global L1 L2 L3;
% q = pi/3;
q = acos((xd(t)^2 + yd(t)^2 +(zd(t)-L3-1.5)^2-L1^2-L2^2)/(2*L1*L2));
% q = 1.57;
end

function y = th3d(t)
L0=1.5;L1=0.3;L2=0.3;L3=0.08; % L3 항상 지면에 수직. 
tf=10; w = 10*pi/tf;
% global L1 L2 L3;
y = pi/2 - th1d(t) - th2d(t);
% y = 1.52;
end

function y = xd(t)
L0=1.5;L1=0.3;L2=0.3;L3=0.08; % L3 항상 지면에 수직.
scale_factor = 1/80; cycle = 1;
tf=10; w = 2*pi*cycle;
y = scale_factor*(6 + cos(w*s(t)))-4.1750e-04- 1.469294361278199e-06;
% global L1 L2 L3 w tf;
% y = ((10 - (10/tf)*(t))*cos(w*(t)))/100;
% y = ((10 - (10/tf)*s(t))*cos(w*s(t)))/100;
% y = (50*cos(pi/4)+(-2*50*cos(pi/4))*s(t)/tf)/100; % 서빙 to 어피치 
end

function y = yd(t)
L0=1.5;L1=0.3;L2=0.3;L3=0.08; % L3 항상 지면에 수직. 
scale_factor = 1/80; cycle = 1;
tf=10; w = 2*pi*cycle;
y = scale_factor*(6+ sin(w*s(t))) + 0.4-1.0582e-04+ 0.00000326818465700;
% global L1 L2 L3 w tf;
% y = ((10 - (10/tf)*(t))*sin(w*(t)) + 40)/100;  % (0,40) 에서 sprial sink./*
% y = ((10 - (10/tf)*s(t))*sin(w*s(t)) + 40)/100;  % (0,40) 에서 sprial sink.
% y = (0.7 .* s(t).*(s(t)-10) + 50*sin(pi/4))/100; % 두배가량 내려감
end

function y = zd(t)
L0=1.5;L1=0.3;L2=0.3;L3=0.08; % L3 항상 지면에 수직. 
scale_factor = 1/80; cycle = 1;
tf=10; w = 2*pi*cycle;
y = 1.3+ 0.000013186867988;
end
